simulink model "Linearhopf_squaretorque_0_5"  (R2019b)
settings: Solver=ode45  StartTime=0.0  StopTime=10  MaxStep=1e-3  RelTol=1e-3  AbsTol=1e-3
model workspace: external: MATLAB File sm_bumper_car_parameters.m (data not in the file)
undefined symbols (not defined in the file): BackLeft, BackRight, car, critical_velocity, damping, FrontLeft, FrontRight, g, kinetic_friction_coef, Link1, Link2, Link3, Link4, Link5, Link6, Link7, Link8, Link9, static_friction_coef, stiffness, transition_region_width, Wheel5, Wheel6, Wheel7, Wheel8, Wheel9, X, Y, Z
libraries: sm_lib x74, nesl_utility x19, sm_bumper_car_lib x9, simulink x7
(part 2 of 2)

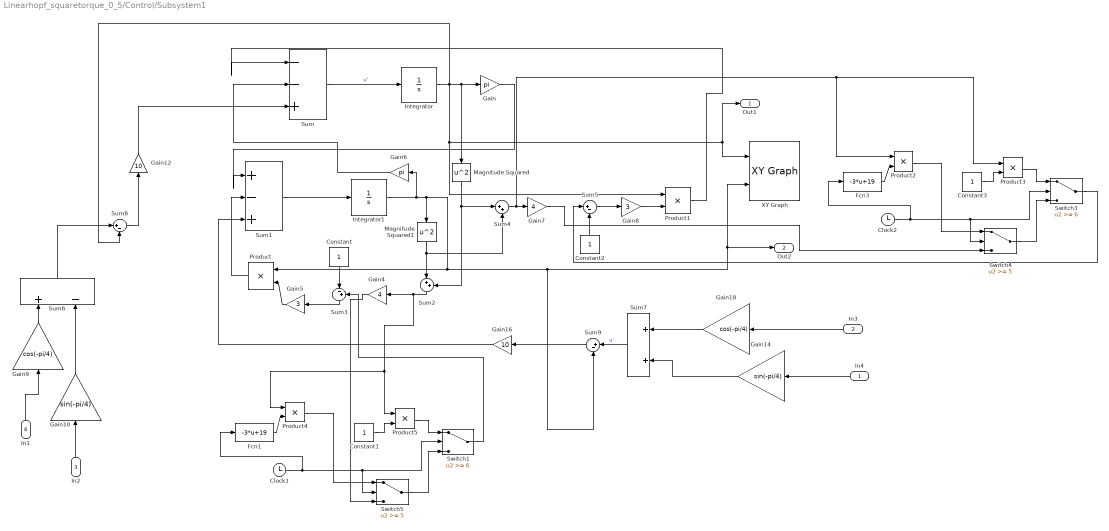
== system Linearhopf_squaretorque_0_5/Control/Subsystem1 ==
  In4 : Inport
  In3 : Inport  Port=2
  In2 : Inport  Port=3
  In1 : Inport  Port=4
  Clock1 : Clock
  Clock2 : Clock
  Constant{,1..3} (4 alike) : Constant
  Fcn1 : Fcn  Expr=-3*u+19
  Fcn3 : Fcn  Expr=-3*u+19
  Gain : Gain  Gain=pi
  Gain10 : Gain  Gain=sin(-pi/4)
  Gain12 : Gain  Gain=10
  Gain14 : Gain  Gain=sin(-pi/4)
  Gain16 : Gain  Gain=10
  Gain18 : Gain  Gain=cos(-pi/4)
  Gain4 : Gain  Gain=4
  Gain5 : Gain  Gain=3
  Gain6 : Gain  Gain=pi
  Gain7 : Gain  Gain=4
  Gain8 : Gain  Gain=3
  Gain9 : Gain  Gain=cos(-pi/4)
  Integrator : Integrator
  Integrator1 : Integrator
  Magnitude Squared : Math  Operator=square  SignedPower=off  SaturateOnIntegerOverflow=on
  Magnitude Squared1 : Math  Operator=square  SignedPower=off  SaturateOnIntegerOverflow=on
  Product{,1..5} (6 alike) : Product
  Sum : Sum  Inputs=|--+
  Sum1 : Sum  Inputs=|+-+
  Sum2 : Sum  Inputs=|++
  Sum3 : Sum  Inputs=|-+
  Sum4 : Sum  Inputs=|++
  Sum5 : Sum  Inputs=|+-
  Sum6 : Sum  Inputs=+-
  Sum7 : Sum
  Sum8 : Sum  Inputs=|+-
  Sum9 : Sum  Inputs=|+-
  Switch1 : Switch  Threshold=6
  Switch3 : Switch  Threshold=6
  Switch4 : Switch  Threshold=5
  Switch5 : Switch  Threshold=5
  XY Graph : simulink/Sinks/XY Graph  xmin=-1  xmax=1  ymin=-1  ymax=1  st=0.01
  Out1 : Outport
  Out2 : Outport  Port=2
  wires:
  Sum1/1 -> Integrator1/1
  Sum/1 -> Integrator/1  "u‘"
  Magnitude Squared/1 -> Sum4/1, Sum2/2
  Product/1 -> Sum1/2
  Constant/1 -> Sum3/1
  Gain6/1 -> Sum/2
  Sum2/1 -> Product4/1, Product5/1, Gain4/1
  Gain/1 -> Sum1/1
  Sum3/1 -> Gain5/1
  Gain5/1 -> Product/2
  Gain8/1 -> Product1/2
  Integrator/1 -> Product1/1, XY Graph/1, Out1/1, Sum8/2, Magnitude Squared/1, Gain/1
  Product1/1 -> Sum/1
  Sum5/1 -> Gain8/1
  Constant2/1 -> Sum5/2
  Magnitude Squared1/1 -> Sum4/2, Sum2/1
  Integrator1/1 -> Product/1, XY Graph/2, Out2/1, Sum9/2, Magnitude Squared1/1, Gain6/1
  Gain9/1 -> Sum6/1
  Gain10/1 -> Sum6/2
  Sum8/1 -> Gain12/1
  Gain12/1 -> Sum/3
  In1/1 -> Gain9/1
  In2/1 -> Gain10/1
  Sum9/1 -> Gain16/1
  Gain14/1 -> Sum7/2
  Gain18/1 -> Sum7/1
  In4/1 -> Gain14/1
  In3/1 -> Gain18/1
  Gain16/1 -> Sum1/3
  Sum7/1 -> Sum9/1  "u‘"
  Sum6/1 -> Sum8/1
  Gain7/1 -> Switch4/3
  Switch5/1 -> Switch1/3
  Clock1/1 -> Fcn1/1, Switch1/2, Switch5/2
  Product5/1 -> Switch1/1
  Fcn1/1 -> Product4/2
  Product4/1 -> Switch5/1
  Constant1/1 -> Product5/2
  Switch1/1 -> Sum3/2
  Gain4/1 -> Switch5/3
  Switch4/1 -> Switch3/3
  Clock2/1 -> Fcn3/1, Switch3/2, Switch4/2
  Product3/1 -> Switch3/1
  Fcn3/1 -> Product2/2
  Product2/1 -> Switch4/1
  Constant3/1 -> Product3/2
  Sum4/1 -> Product3/1, Product2/1, Gain7/1
  Switch3/1 -> Sum5/1

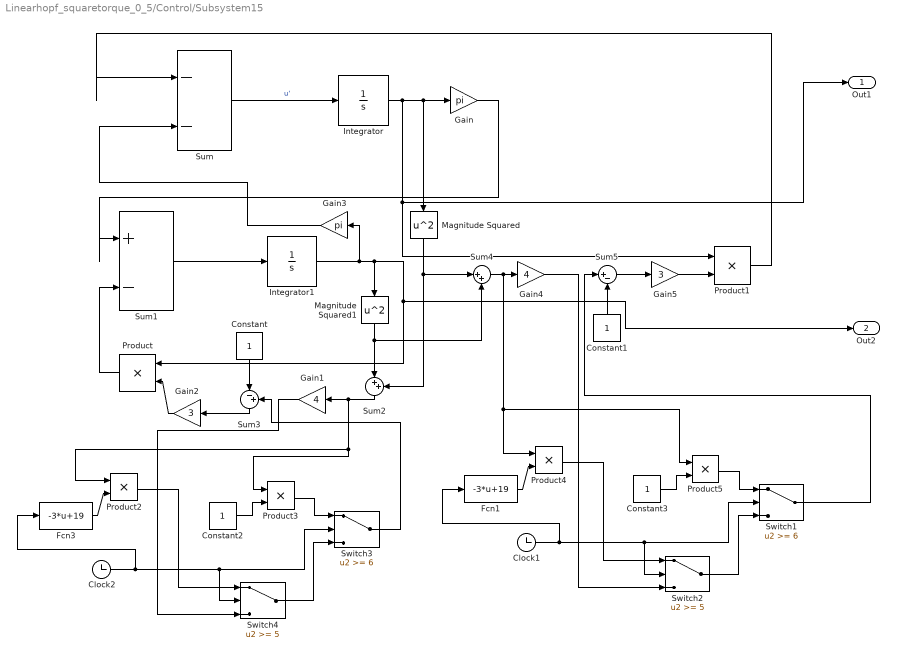
== system Linearhopf_squaretorque_0_5/Control/Subsystem15 ==
  Clock1 : Clock
  Clock2 : Clock
  Constant{,1..3} (4 alike) : Constant
  Fcn1 : Fcn  Expr=-3*u+19
  Fcn3 : Fcn  Expr=-3*u+19
  Gain : Gain  Gain=pi
  Gain1 : Gain  Gain=4
  Gain2 : Gain  Gain=3
  Gain3 : Gain  Gain=pi
  Gain4 : Gain  Gain=4
  Gain5 : Gain  Gain=3
  Integrator : Integrator  InitialCondition=0.01
  Integrator1 : Integrator
  Magnitude Squared : Math  Operator=square  SignedPower=off  SaturateOnIntegerOverflow=on
  Magnitude Squared1 : Math  Operator=square  SignedPower=off  SaturateOnIntegerOverflow=on
  Product{,1..5} (6 alike) : Product
  Sum : Sum  Inputs=|--
  Sum1 : Sum  Inputs=|+-
  Sum2 : Sum  Inputs=|++
  Sum3 : Sum  Inputs=|-+
  Sum4 : Sum  Inputs=|++
  Sum5 : Sum  Inputs=|+-
  Switch1 : Switch  Threshold=6
  Switch2 : Switch  Threshold=5
  Switch3 : Switch  Threshold=6
  Switch4 : Switch  Threshold=5
  Out1 : Outport
  Out2 : Outport  Port=2
  wires:
  Integrator1/1 -> Product/1, Out2/1, Magnitude Squared1/1, Gain3/1
  Sum5/1 -> Gain5/1
  Constant1/1 -> Sum5/2
  Product1/1 -> Sum/1
  Magnitude Squared1/1 -> Sum4/2, Sum2/1
  Gain2/1 -> Product/2
  Sum3/1 -> Gain2/1
  Gain/1 -> Sum1/1
  Gain5/1 -> Product1/2
  Integrator/1 -> Product1/1, Out1/1, Magnitude Squared/1, Gain/1
  Product/1 -> Sum1/2
  Sum2/1 -> Product3/1, Product2/1, Gain1/1
  Constant/1 -> Sum3/1
  Magnitude Squared/1 -> Sum4/1, Sum2/2
  Gain3/1 -> Sum/2
  Sum1/1 -> Integrator1/1
  Sum/1 -> Integrator/1  "u‘"
  Sum4/1 -> Product4/1, Product5/1, Gain4/1
  Clock2/1 -> Fcn3/1, Switch3/2, Switch4/2
  Switch4/1 -> Switch3/3
  Fcn3/1 -> Product2/2
  Product2/1 -> Switch4/1
  Gain1/1 -> Switch4/3
  Constant2/1 -> Product3/2
  Switch3/1 -> Sum3/2
  Product3/1 -> Switch3/1
  Switch2/1 -> Switch1/3
  Clock1/1 -> Fcn1/1, Switch1/2, Switch2/2
  Product5/1 -> Switch1/1
  Switch1/1 -> Sum5/1
  Fcn1/1 -> Product4/2
  Product4/1 -> Switch2/1
  Constant3/1 -> Product5/2
  Gain4/1 -> Switch2/3

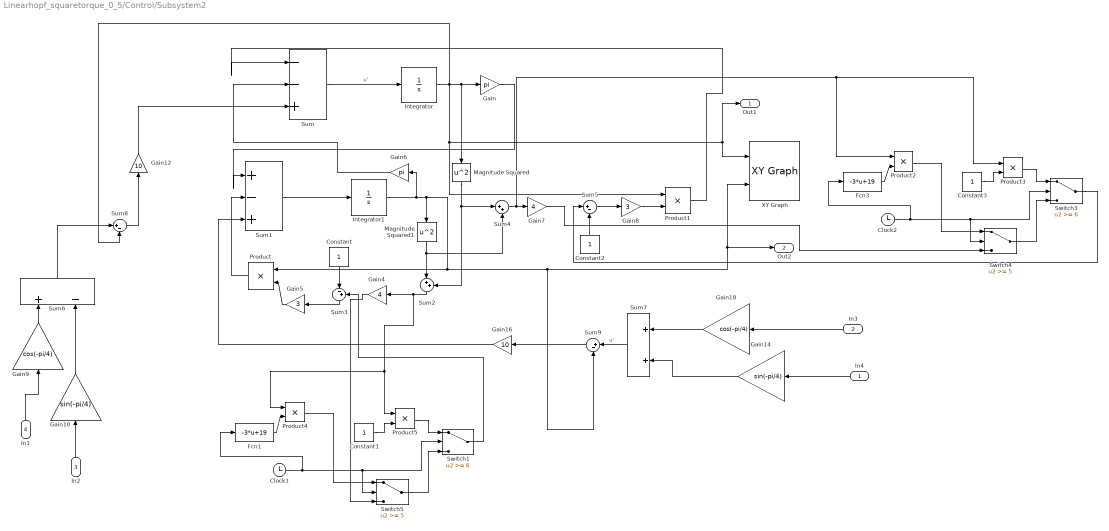
== system Linearhopf_squaretorque_0_5/Control/Subsystem2 ==
  In4 : Inport
  In3 : Inport  Port=2
  In2 : Inport  Port=3
  In1 : Inport  Port=4
  Clock1 : Clock
  Clock2 : Clock
  Constant{,1..3} (4 alike) : Constant
  Fcn1 : Fcn  Expr=-3*u+19
  Fcn3 : Fcn  Expr=-3*u+19
  Gain : Gain  Gain=pi
  Gain10 : Gain  Gain=sin(-pi/4)
  Gain12 : Gain  Gain=10
  Gain14 : Gain  Gain=sin(-pi/4)
  Gain16 : Gain  Gain=10
  Gain18 : Gain  Gain=cos(-pi/4)
  Gain4 : Gain  Gain=4
  Gain5 : Gain  Gain=3
  Gain6 : Gain  Gain=pi
  Gain7 : Gain  Gain=4
  Gain8 : Gain  Gain=3
  Gain9 : Gain  Gain=cos(-pi/4)
  Integrator : Integrator
  Integrator1 : Integrator
  Magnitude Squared : Math  Operator=square  SignedPower=off  SaturateOnIntegerOverflow=on
  Magnitude Squared1 : Math  Operator=square  SignedPower=off  SaturateOnIntegerOverflow=on
  Product{,1..5} (6 alike) : Product
  Sum : Sum  Inputs=|--+
  Sum1 : Sum  Inputs=|+-+
  Sum2 : Sum  Inputs=|++
  Sum3 : Sum  Inputs=|-+
  Sum4 : Sum  Inputs=|++
  Sum5 : Sum  Inputs=|+-
  Sum6 : Sum  Inputs=+-
  Sum7 : Sum
  Sum8 : Sum  Inputs=|+-
  Sum9 : Sum  Inputs=|+-
  Switch1 : Switch  Threshold=6
  Switch3 : Switch  Threshold=6
  Switch4 : Switch  Threshold=5
  Switch5 : Switch  Threshold=5
  XY Graph : simulink/Sinks/XY Graph  xmin=-1  xmax=1  ymin=-1  ymax=1  st=0.01
  Out1 : Outport
  Out2 : Outport  Port=2
  wires:
  Sum1/1 -> Integrator1/1
  Sum/1 -> Integrator/1  "u‘"
  Magnitude Squared/1 -> Sum4/1, Sum2/2
  Product/1 -> Sum1/2
  Constant/1 -> Sum3/1
  Gain6/1 -> Sum/2
  Sum2/1 -> Product4/1, Product5/1, Gain4/1
  Gain/1 -> Sum1/1
  Sum3/1 -> Gain5/1
  Gain5/1 -> Product/2
  Gain8/1 -> Product1/2
  Integrator/1 -> Product1/1, XY Graph/1, Out1/1, Sum8/2, Magnitude Squared/1, Gain/1
  Product1/1 -> Sum/1
  Sum5/1 -> Gain8/1
  Constant2/1 -> Sum5/2
  Magnitude Squared1/1 -> Sum4/2, Sum2/1
  Integrator1/1 -> Product/1, XY Graph/2, Out2/1, Sum9/2, Magnitude Squared1/1, Gain6/1
  Gain9/1 -> Sum6/1
  Gain10/1 -> Sum6/2
  Sum8/1 -> Gain12/1
  Gain12/1 -> Sum/3
  In1/1 -> Gain9/1
  In2/1 -> Gain10/1
  Sum9/1 -> Gain16/1
  Gain14/1 -> Sum7/2
  Gain18/1 -> Sum7/1
  In4/1 -> Gain14/1
  In3/1 -> Gain18/1
  Gain16/1 -> Sum1/3
  Sum7/1 -> Sum9/1  "u‘"
  Sum6/1 -> Sum8/1
  Gain7/1 -> Switch4/3
  Switch5/1 -> Switch1/3
  Clock1/1 -> Fcn1/1, Switch1/2, Switch5/2
  Product5/1 -> Switch1/1
  Fcn1/1 -> Product4/2
  Product4/1 -> Switch5/1
  Constant1/1 -> Product5/2
  Switch1/1 -> Sum3/2
  Gain4/1 -> Switch5/3
  Switch4/1 -> Switch3/3
  Clock2/1 -> Fcn3/1, Switch3/2, Switch4/2
  Product3/1 -> Switch3/1
  Fcn3/1 -> Product2/2
  Product2/1 -> Switch4/1
  Constant3/1 -> Product3/2
  Sum4/1 -> Product3/1, Product2/1, Gain7/1
  Switch3/1 -> Sum5/1

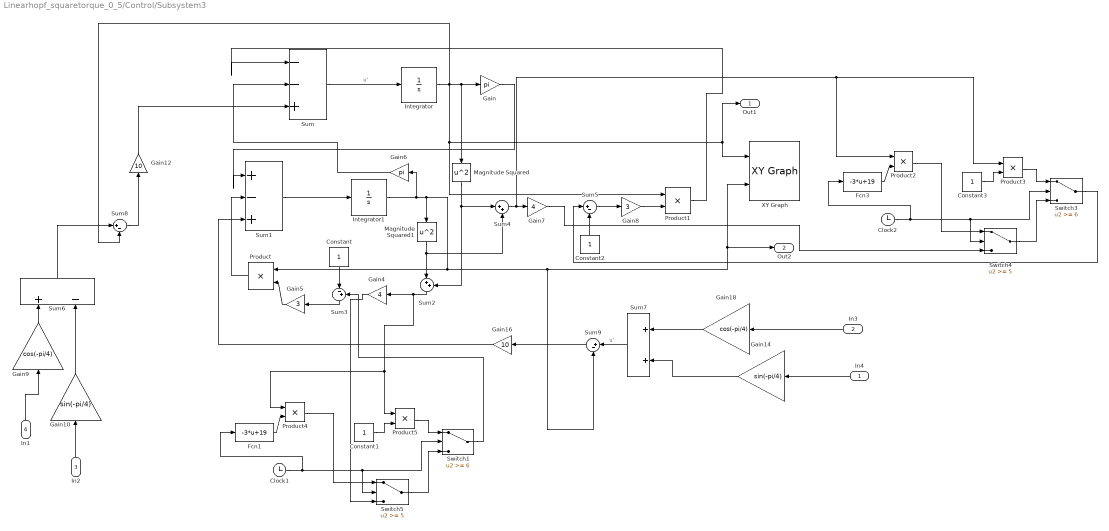
== system Linearhopf_squaretorque_0_5/Control/Subsystem3 ==
  In4 : Inport
  In3 : Inport  Port=2
  In2 : Inport  Port=3
  In1 : Inport  Port=4
  Clock1 : Clock
  Clock2 : Clock
  Constant{,1..3} (4 alike) : Constant
  Fcn1 : Fcn  Expr=-3*u+19
  Fcn3 : Fcn  Expr=-3*u+19
  Gain : Gain  Gain=pi
  Gain10 : Gain  Gain=sin(-pi/4)
  Gain12 : Gain  Gain=10
  Gain14 : Gain  Gain=sin(-pi/4)
  Gain16 : Gain  Gain=10
  Gain18 : Gain  Gain=cos(-pi/4)
  Gain4 : Gain  Gain=4
  Gain5 : Gain  Gain=3
  Gain6 : Gain  Gain=pi
  Gain7 : Gain  Gain=4
  Gain8 : Gain  Gain=3
  Gain9 : Gain  Gain=cos(-pi/4)
  Integrator : Integrator
  Integrator1 : Integrator
  Magnitude Squared : Math  Operator=square  SignedPower=off  SaturateOnIntegerOverflow=on
  Magnitude Squared1 : Math  Operator=square  SignedPower=off  SaturateOnIntegerOverflow=on
  Product{,1..5} (6 alike) : Product
  Sum : Sum  Inputs=|--+
  Sum1 : Sum  Inputs=|+-+
  Sum2 : Sum  Inputs=|++
  Sum3 : Sum  Inputs=|-+
  Sum4 : Sum  Inputs=|++
  Sum5 : Sum  Inputs=|+-
  Sum6 : Sum  Inputs=+-
  Sum7 : Sum
  Sum8 : Sum  Inputs=|+-
  Sum9 : Sum  Inputs=|+-
  Switch1 : Switch  Threshold=6
  Switch3 : Switch  Threshold=6
  Switch4 : Switch  Threshold=5
  Switch5 : Switch  Threshold=5
  XY Graph : simulink/Sinks/XY Graph  xmin=-1  xmax=1  ymin=-1  ymax=1  st=0.01
  Out1 : Outport
  Out2 : Outport  Port=2
  wires:
  Sum1/1 -> Integrator1/1
  Sum/1 -> Integrator/1  "u‘"
  Magnitude Squared/1 -> Sum4/1, Sum2/2
  Product/1 -> Sum1/2
  Constant/1 -> Sum3/1
  Gain6/1 -> Sum/2
  Sum2/1 -> Product4/1, Product5/1, Gain4/1
  Gain/1 -> Sum1/1
  Sum3/1 -> Gain5/1
  Gain5/1 -> Product/2
  Gain8/1 -> Product1/2
  Integrator/1 -> Product1/1, XY Graph/1, Out1/1, Sum8/2, Magnitude Squared/1, Gain/1
  Product1/1 -> Sum/1
  Sum5/1 -> Gain8/1
  Constant2/1 -> Sum5/2
  Magnitude Squared1/1 -> Sum4/2, Sum2/1
  Integrator1/1 -> Product/1, XY Graph/2, Out2/1, Sum9/2, Magnitude Squared1/1, Gain6/1
  Gain9/1 -> Sum6/1
  Gain10/1 -> Sum6/2
  Sum8/1 -> Gain12/1
  Gain12/1 -> Sum/3
  In1/1 -> Gain9/1
  In2/1 -> Gain10/1
  Sum9/1 -> Gain16/1
  Gain14/1 -> Sum7/2
  Gain18/1 -> Sum7/1
  In4/1 -> Gain14/1
  In3/1 -> Gain18/1
  Gain16/1 -> Sum1/3
  Sum7/1 -> Sum9/1  "u‘"
  Sum6/1 -> Sum8/1
  Gain7/1 -> Switch4/3
  Switch5/1 -> Switch1/3
  Clock1/1 -> Fcn1/1, Switch1/2, Switch5/2
  Product5/1 -> Switch1/1
  Fcn1/1 -> Product4/2
  Product4/1 -> Switch5/1
  Constant1/1 -> Product5/2
  Switch1/1 -> Sum3/2
  Gain4/1 -> Switch5/3
  Switch4/1 -> Switch3/3
  Clock2/1 -> Fcn3/1, Switch3/2, Switch4/2
  Product3/1 -> Switch3/1
  Fcn3/1 -> Product2/2
  Product2/1 -> Switch4/1
  Constant3/1 -> Product3/2
  Sum4/1 -> Product3/1, Product2/1, Gain7/1
  Switch3/1 -> Sum5/1

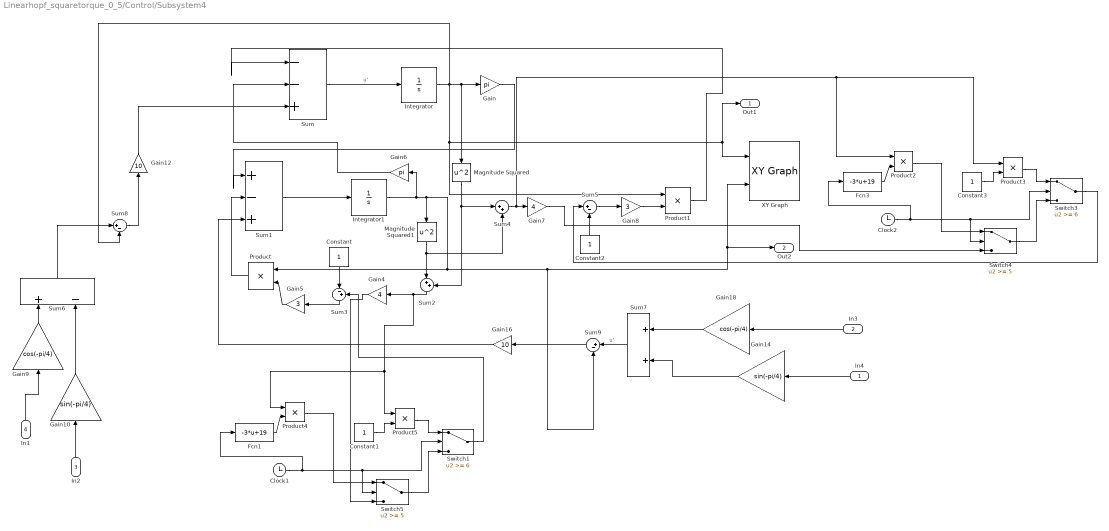
== system Linearhopf_squaretorque_0_5/Control/Subsystem4 ==
  In4 : Inport
  In3 : Inport  Port=2
  In2 : Inport  Port=3
  In1 : Inport  Port=4
  Clock1 : Clock
  Clock2 : Clock
  Constant{,1..3} (4 alike) : Constant
  Fcn1 : Fcn  Expr=-3*u+19
  Fcn3 : Fcn  Expr=-3*u+19
  Gain : Gain  Gain=pi
  Gain10 : Gain  Gain=sin(-pi/4)
  Gain12 : Gain  Gain=10
  Gain14 : Gain  Gain=sin(-pi/4)
  Gain16 : Gain  Gain=10
  Gain18 : Gain  Gain=cos(-pi/4)
  Gain4 : Gain  Gain=4
  Gain5 : Gain  Gain=3
  Gain6 : Gain  Gain=pi
  Gain7 : Gain  Gain=4
  Gain8 : Gain  Gain=3
  Gain9 : Gain  Gain=cos(-pi/4)
  Integrator : Integrator
  Integrator1 : Integrator
  Magnitude Squared : Math  Operator=square  SignedPower=off  SaturateOnIntegerOverflow=on
  Magnitude Squared1 : Math  Operator=square  SignedPower=off  SaturateOnIntegerOverflow=on
  Product{,1..5} (6 alike) : Product
  Sum : Sum  Inputs=|--+
  Sum1 : Sum  Inputs=|+-+
  Sum2 : Sum  Inputs=|++
  Sum3 : Sum  Inputs=|-+
  Sum4 : Sum  Inputs=|++
  Sum5 : Sum  Inputs=|+-
  Sum6 : Sum  Inputs=+-
  Sum7 : Sum
  Sum8 : Sum  Inputs=|+-
  Sum9 : Sum  Inputs=|+-
  Switch1 : Switch  Threshold=6
  Switch3 : Switch  Threshold=6
  Switch4 : Switch  Threshold=5
  Switch5 : Switch  Threshold=5
  XY Graph : simulink/Sinks/XY Graph  xmin=-1  xmax=1  ymin=-1  ymax=1  st=0.01
  Out1 : Outport
  Out2 : Outport  Port=2
  wires:
  Sum1/1 -> Integrator1/1
  Sum/1 -> Integrator/1  "u‘"
  Magnitude Squared/1 -> Sum4/1, Sum2/2
  Product/1 -> Sum1/2
  Constant/1 -> Sum3/1
  Gain6/1 -> Sum/2
  Sum2/1 -> Product4/1, Product5/1, Gain4/1
  Gain/1 -> Sum1/1
  Sum3/1 -> Gain5/1
  Gain5/1 -> Product/2
  Gain8/1 -> Product1/2
  Integrator/1 -> Product1/1, XY Graph/1, Out1/1, Sum8/2, Magnitude Squared/1, Gain/1
  Product1/1 -> Sum/1
  Sum5/1 -> Gain8/1
  Constant2/1 -> Sum5/2
  Magnitude Squared1/1 -> Sum4/2, Sum2/1
  Integrator1/1 -> Product/1, XY Graph/2, Out2/1, Sum9/2, Magnitude Squared1/1, Gain6/1
  Gain9/1 -> Sum6/1
  Gain10/1 -> Sum6/2
  Sum8/1 -> Gain12/1
  Gain12/1 -> Sum/3
  In1/1 -> Gain9/1
  In2/1 -> Gain10/1
  Sum9/1 -> Gain16/1
  Gain14/1 -> Sum7/2
  Gain18/1 -> Sum7/1
  In4/1 -> Gain14/1
  In3/1 -> Gain18/1
  Gain16/1 -> Sum1/3
  Sum7/1 -> Sum9/1  "u‘"
  Sum6/1 -> Sum8/1
  Gain7/1 -> Switch4/3
  Switch5/1 -> Switch1/3
  Clock1/1 -> Fcn1/1, Switch1/2, Switch5/2
  Product5/1 -> Switch1/1
  Fcn1/1 -> Product4/2
  Product4/1 -> Switch5/1
  Constant1/1 -> Product5/2
  Switch1/1 -> Sum3/2
  Gain4/1 -> Switch5/3
  Switch4/1 -> Switch3/3
  Clock2/1 -> Fcn3/1, Switch3/2, Switch4/2
  Product3/1 -> Switch3/1
  Fcn3/1 -> Product2/2
  Product2/1 -> Switch4/1
  Constant3/1 -> Product3/2
  Sum4/1 -> Product3/1, Product2/1, Gain7/1
  Switch3/1 -> Sum5/1

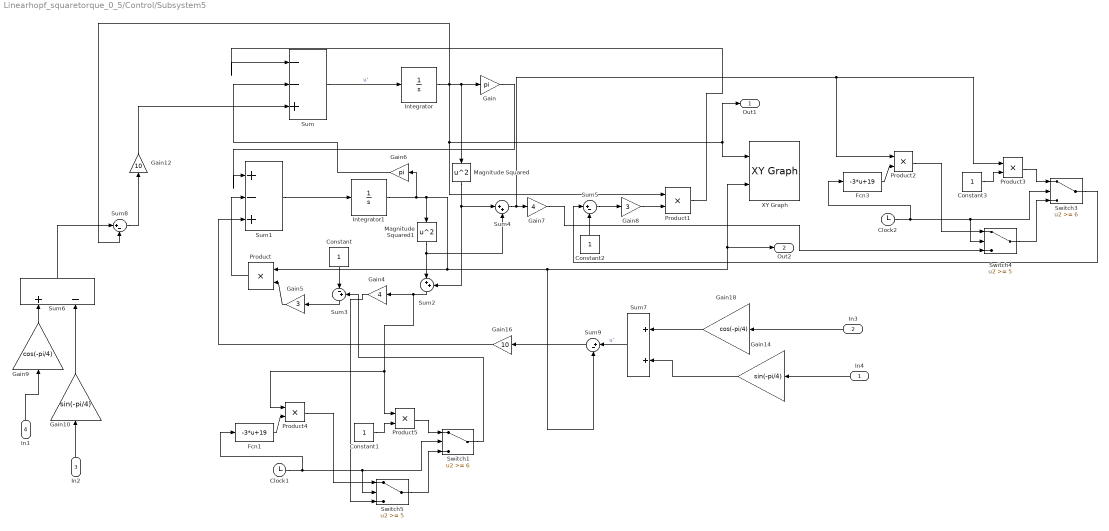
== system Linearhopf_squaretorque_0_5/Control/Subsystem5 ==
  In4 : Inport
  In3 : Inport  Port=2
  In2 : Inport  Port=3
  In1 : Inport  Port=4
  Clock1 : Clock
  Clock2 : Clock
  Constant{,1..3} (4 alike) : Constant
  Fcn1 : Fcn  Expr=-3*u+19
  Fcn3 : Fcn  Expr=-3*u+19
  Gain : Gain  Gain=pi
  Gain10 : Gain  Gain=sin(-pi/4)
  Gain12 : Gain  Gain=10
  Gain14 : Gain  Gain=sin(-pi/4)
  Gain16 : Gain  Gain=10
  Gain18 : Gain  Gain=cos(-pi/4)
  Gain4 : Gain  Gain=4
  Gain5 : Gain  Gain=3
  Gain6 : Gain  Gain=pi
  Gain7 : Gain  Gain=4
  Gain8 : Gain  Gain=3
  Gain9 : Gain  Gain=cos(-pi/4)
  Integrator : Integrator
  Integrator1 : Integrator
  Magnitude Squared : Math  Operator=square  SignedPower=off  SaturateOnIntegerOverflow=on
  Magnitude Squared1 : Math  Operator=square  SignedPower=off  SaturateOnIntegerOverflow=on
  Product{,1..5} (6 alike) : Product
  Sum : Sum  Inputs=|--+
  Sum1 : Sum  Inputs=|+-+
  Sum2 : Sum  Inputs=|++
  Sum3 : Sum  Inputs=|-+
  Sum4 : Sum  Inputs=|++
  Sum5 : Sum  Inputs=|+-
  Sum6 : Sum  Inputs=+-
  Sum7 : Sum
  Sum8 : Sum  Inputs=|+-
  Sum9 : Sum  Inputs=|+-
  Switch1 : Switch  Threshold=6
  Switch3 : Switch  Threshold=6
  Switch4 : Switch  Threshold=5
  Switch5 : Switch  Threshold=5
  XY Graph : simulink/Sinks/XY Graph  xmin=-1  xmax=1  ymin=-1  ymax=1  st=0.01
  Out1 : Outport
  Out2 : Outport  Port=2
  wires:
  Sum1/1 -> Integrator1/1
  Sum/1 -> Integrator/1  "u‘"
  Magnitude Squared/1 -> Sum4/1, Sum2/2
  Product/1 -> Sum1/2
  Constant/1 -> Sum3/1
  Gain6/1 -> Sum/2
  Sum2/1 -> Product4/1, Product5/1, Gain4/1
  Gain/1 -> Sum1/1
  Sum3/1 -> Gain5/1
  Gain5/1 -> Product/2
  Gain8/1 -> Product1/2
  Integrator/1 -> Product1/1, XY Graph/1, Out1/1, Sum8/2, Magnitude Squared/1, Gain/1
  Product1/1 -> Sum/1
  Sum5/1 -> Gain8/1
  Constant2/1 -> Sum5/2
  Magnitude Squared1/1 -> Sum4/2, Sum2/1
  Integrator1/1 -> Product/1, XY Graph/2, Out2/1, Sum9/2, Magnitude Squared1/1, Gain6/1
  Gain9/1 -> Sum6/1
  Gain10/1 -> Sum6/2
  Sum8/1 -> Gain12/1
  Gain12/1 -> Sum/3
  In1/1 -> Gain9/1
  In2/1 -> Gain10/1
  Sum9/1 -> Gain16/1
  Gain14/1 -> Sum7/2
  Gain18/1 -> Sum7/1
  In4/1 -> Gain14/1
  In3/1 -> Gain18/1
  Gain16/1 -> Sum1/3
  Sum7/1 -> Sum9/1  "u‘"
  Sum6/1 -> Sum8/1
  Gain7/1 -> Switch4/3
  Switch5/1 -> Switch1/3
  Clock1/1 -> Fcn1/1, Switch1/2, Switch5/2
  Product5/1 -> Switch1/1
  Fcn1/1 -> Product4/2
  Product4/1 -> Switch5/1
  Constant1/1 -> Product5/2
  Switch1/1 -> Sum3/2
  Gain4/1 -> Switch5/3
  Switch4/1 -> Switch3/3
  Clock2/1 -> Fcn3/1, Switch3/2, Switch4/2
  Product3/1 -> Switch3/1
  Fcn3/1 -> Product2/2
  Product2/1 -> Switch4/1
  Constant3/1 -> Product3/2
  Sum4/1 -> Product3/1, Product2/1, Gain7/1
  Switch3/1 -> Sum5/1

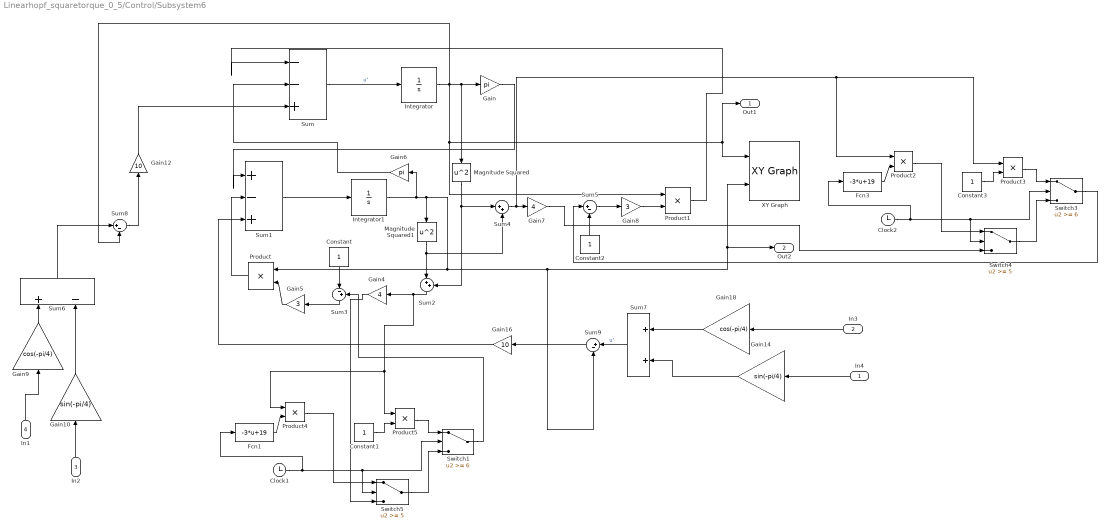
== system Linearhopf_squaretorque_0_5/Control/Subsystem6 ==
  In4 : Inport
  In3 : Inport  Port=2
  In2 : Inport  Port=3
  In1 : Inport  Port=4
  Clock1 : Clock
  Clock2 : Clock
  Constant{,1..3} (4 alike) : Constant
  Fcn1 : Fcn  Expr=-3*u+19
  Fcn3 : Fcn  Expr=-3*u+19
  Gain : Gain  Gain=pi
  Gain10 : Gain  Gain=sin(-pi/4)
  Gain12 : Gain  Gain=10
  Gain14 : Gain  Gain=sin(-pi/4)
  Gain16 : Gain  Gain=10
  Gain18 : Gain  Gain=cos(-pi/4)
  Gain4 : Gain  Gain=4
  Gain5 : Gain  Gain=3
  Gain6 : Gain  Gain=pi
  Gain7 : Gain  Gain=4
  Gain8 : Gain  Gain=3
  Gain9 : Gain  Gain=cos(-pi/4)
  Integrator : Integrator
  Integrator1 : Integrator
  Magnitude Squared : Math  Operator=square  SignedPower=off  SaturateOnIntegerOverflow=on
  Magnitude Squared1 : Math  Operator=square  SignedPower=off  SaturateOnIntegerOverflow=on
  Product{,1..5} (6 alike) : Product
  Sum : Sum  Inputs=|--+
  Sum1 : Sum  Inputs=|+-+
  Sum2 : Sum  Inputs=|++
  Sum3 : Sum  Inputs=|-+
  Sum4 : Sum  Inputs=|++
  Sum5 : Sum  Inputs=|+-
  Sum6 : Sum  Inputs=+-
  Sum7 : Sum
  Sum8 : Sum  Inputs=|+-
  Sum9 : Sum  Inputs=|+-
  Switch1 : Switch  Threshold=6
  Switch3 : Switch  Threshold=6
  Switch4 : Switch  Threshold=5
  Switch5 : Switch  Threshold=5
  XY Graph : simulink/Sinks/XY Graph  xmin=-1  xmax=1  ymin=-1  ymax=1  st=0.01
  Out1 : Outport
  Out2 : Outport  Port=2
  wires:
  Sum1/1 -> Integrator1/1
  Sum/1 -> Integrator/1  "u‘"
  Magnitude Squared/1 -> Sum4/1, Sum2/2
  Product/1 -> Sum1/2
  Constant/1 -> Sum3/1
  Gain6/1 -> Sum/2
  Sum2/1 -> Product4/1, Product5/1, Gain4/1
  Gain/1 -> Sum1/1
  Sum3/1 -> Gain5/1
  Gain5/1 -> Product/2
  Gain8/1 -> Product1/2
  Integrator/1 -> Product1/1, XY Graph/1, Out1/1, Sum8/2, Magnitude Squared/1, Gain/1
  Product1/1 -> Sum/1
  Sum5/1 -> Gain8/1
  Constant2/1 -> Sum5/2
  Magnitude Squared1/1 -> Sum4/2, Sum2/1
  Integrator1/1 -> Product/1, XY Graph/2, Out2/1, Sum9/2, Magnitude Squared1/1, Gain6/1
  Gain9/1 -> Sum6/1
  Gain10/1 -> Sum6/2
  Sum8/1 -> Gain12/1
  Gain12/1 -> Sum/3
  In1/1 -> Gain9/1
  In2/1 -> Gain10/1
  Sum9/1 -> Gain16/1
  Gain14/1 -> Sum7/2
  Gain18/1 -> Sum7/1
  In4/1 -> Gain14/1
  In3/1 -> Gain18/1
  Gain16/1 -> Sum1/3
  Sum7/1 -> Sum9/1  "u‘"
  Sum6/1 -> Sum8/1
  Gain7/1 -> Switch4/3
  Switch5/1 -> Switch1/3
  Clock1/1 -> Fcn1/1, Switch1/2, Switch5/2
  Product5/1 -> Switch1/1
  Fcn1/1 -> Product4/2
  Product4/1 -> Switch5/1
  Constant1/1 -> Product5/2
  Switch1/1 -> Sum3/2
  Gain4/1 -> Switch5/3
  Switch4/1 -> Switch3/3
  Clock2/1 -> Fcn3/1, Switch3/2, Switch4/2
  Product3/1 -> Switch3/1
  Fcn3/1 -> Product2/2
  Product2/1 -> Switch4/1
  Constant3/1 -> Product3/2
  Sum4/1 -> Product3/1, Product2/1, Gain7/1
  Switch3/1 -> Sum5/1

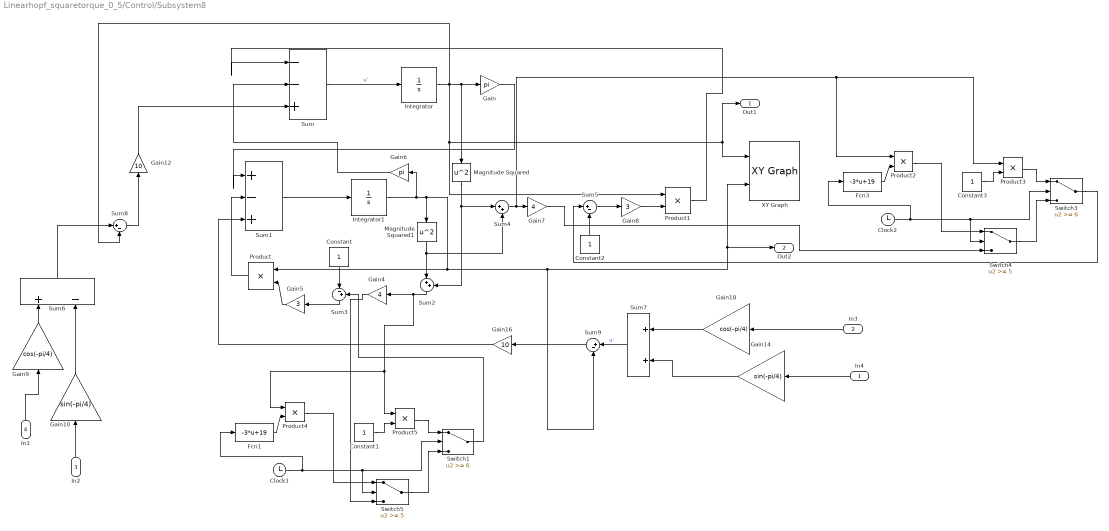
== system Linearhopf_squaretorque_0_5/Control/Subsystem8 ==
  In4 : Inport
  In3 : Inport  Port=2
  In2 : Inport  Port=3
  In1 : Inport  Port=4
  Clock1 : Clock
  Clock2 : Clock
  Constant{,1..3} (4 alike) : Constant
  Fcn1 : Fcn  Expr=-3*u+19
  Fcn3 : Fcn  Expr=-3*u+19
  Gain : Gain  Gain=pi
  Gain10 : Gain  Gain=sin(-pi/4)
  Gain12 : Gain  Gain=10
  Gain14 : Gain  Gain=sin(-pi/4)
  Gain16 : Gain  Gain=10
  Gain18 : Gain  Gain=cos(-pi/4)
  Gain4 : Gain  Gain=4
  Gain5 : Gain  Gain=3
  Gain6 : Gain  Gain=pi
  Gain7 : Gain  Gain=4
  Gain8 : Gain  Gain=3
  Gain9 : Gain  Gain=cos(-pi/4)
  Integrator : Integrator
  Integrator1 : Integrator
  Magnitude Squared : Math  Operator=square  SignedPower=off  SaturateOnIntegerOverflow=on
  Magnitude Squared1 : Math  Operator=square  SignedPower=off  SaturateOnIntegerOverflow=on
  Product{,1..5} (6 alike) : Product
  Sum : Sum  Inputs=|--+
  Sum1 : Sum  Inputs=|+-+
  Sum2 : Sum  Inputs=|++
  Sum3 : Sum  Inputs=|-+
  Sum4 : Sum  Inputs=|++
  Sum5 : Sum  Inputs=|+-
  Sum6 : Sum  Inputs=+-
  Sum7 : Sum
  Sum8 : Sum  Inputs=|+-
  Sum9 : Sum  Inputs=|+-
  Switch1 : Switch  Threshold=6
  Switch3 : Switch  Threshold=6
  Switch4 : Switch  Threshold=5
  Switch5 : Switch  Threshold=5
  XY Graph : simulink/Sinks/XY Graph  xmin=-1  xmax=1  ymin=-1  ymax=1  st=0.01
  Out1 : Outport
  Out2 : Outport  Port=2
  wires:
  Sum1/1 -> Integrator1/1
  Sum/1 -> Integrator/1  "u‘"
  Magnitude Squared/1 -> Sum4/1, Sum2/2
  Product/1 -> Sum1/2
  Constant/1 -> Sum3/1
  Gain6/1 -> Sum/2
  Sum2/1 -> Product4/1, Product5/1, Gain4/1
  Gain/1 -> Sum1/1
  Sum3/1 -> Gain5/1
  Gain5/1 -> Product/2
  Gain8/1 -> Product1/2
  Integrator/1 -> Product1/1, XY Graph/1, Out1/1, Sum8/2, Magnitude Squared/1, Gain/1
  Product1/1 -> Sum/1
  Sum5/1 -> Gain8/1
  Constant2/1 -> Sum5/2
  Magnitude Squared1/1 -> Sum4/2, Sum2/1
  Integrator1/1 -> Product/1, XY Graph/2, Out2/1, Sum9/2, Magnitude Squared1/1, Gain6/1
  Gain9/1 -> Sum6/1
  Gain10/1 -> Sum6/2
  Sum8/1 -> Gain12/1
  Gain12/1 -> Sum/3
  In1/1 -> Gain9/1
  In2/1 -> Gain10/1
  Sum9/1 -> Gain16/1
  Gain14/1 -> Sum7/2
  Gain18/1 -> Sum7/1
  In4/1 -> Gain14/1
  In3/1 -> Gain18/1
  Gain16/1 -> Sum1/3
  Sum7/1 -> Sum9/1  "u‘"
  Sum6/1 -> Sum8/1
  Gain7/1 -> Switch4/3
  Switch5/1 -> Switch1/3
  Clock1/1 -> Fcn1/1, Switch1/2, Switch5/2
  Product5/1 -> Switch1/1
  Fcn1/1 -> Product4/2
  Product4/1 -> Switch5/1
  Constant1/1 -> Product5/2
  Switch1/1 -> Sum3/2
  Gain4/1 -> Switch5/3
  Switch4/1 -> Switch3/3
  Clock2/1 -> Fcn3/1, Switch3/2, Switch4/2
  Product3/1 -> Switch3/1
  Fcn3/1 -> Product2/2
  Product2/1 -> Switch4/1
  Constant3/1 -> Product3/2
  Sum4/1 -> Product3/1, Product2/1, Gain7/1
  Switch3/1 -> Sum5/1
